simulink model "microarchi_router"  (R2015a)
settings: Solver=ode45  StartTime=0.0  StopTime=10.0  RelTol=1e-3
undefined symbols (not defined in the file or in its folder): des
(part 1 of 2)
settings Model: Creator=Nejib  LastModifiedBy=Nejib

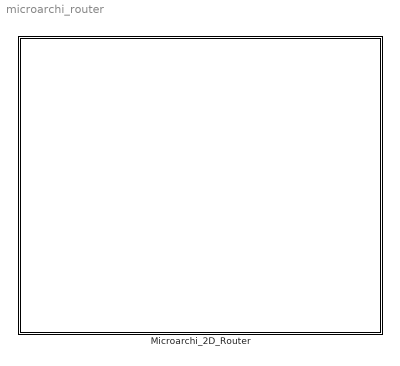
== system microarchi_router ==
  Microarchi_2D_Router : Subsystem  mask{C=16, P=1, ME_X=1, ME_Y=1, N_X=4, N_Y=4}
      mask prompts: C "FIFO size"; P "Clock period"; ME_X "X"; ME_Y "Y"; N_X "X"; N_Y "Y"

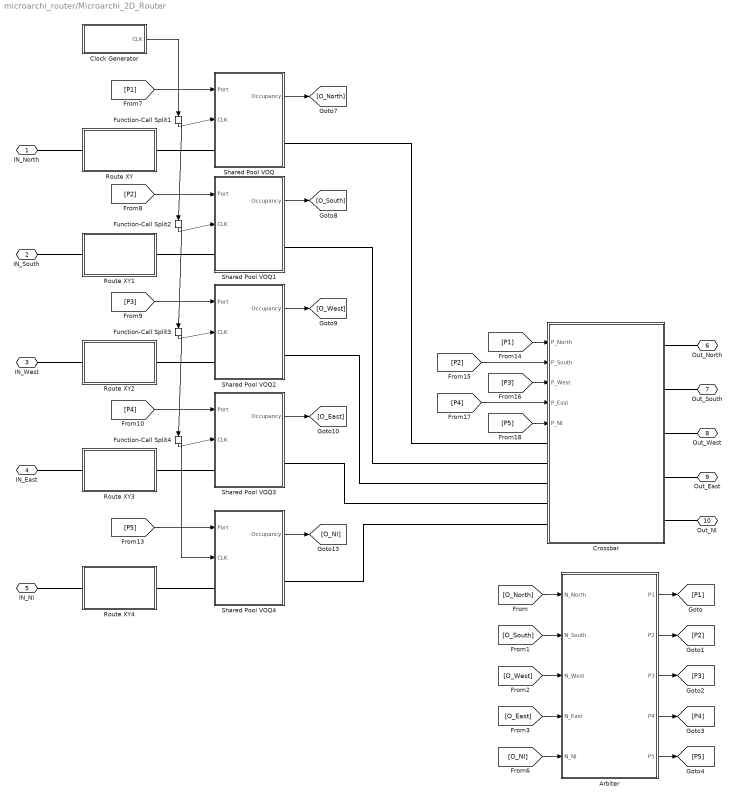
== system microarchi_router/Microarchi_2D_Router ==
  Arbiter : Subsystem  TreatAsAtomicUnit=on
  Clock Generator : Subsystem  mask{P=P}
      mask prompts: P "Period"
      mask DialogControl DescTextVar Prompt: Generates a perfectly periodic clock signal.
  Crossbar : Subsystem
  Function-Call Split{1..4} (4 alike) : FunctionCallSplit
  Route XY : Subsystem  mask{ME_X=ME_X, ME_Y=ME_Y, N_X=4, N_Y=4}
      mask prompts: ME_X "X"; ME_Y "Y"; N_X "X"; N_Y "Y"
  Route XY1 : Subsystem  mask{ME_X=ME_X, ME_Y=ME_Y, N_X=4, N_Y=4}
      mask prompts: ME_X "X"; ME_Y "Y"; N_X "X"; N_Y "Y"
  Route XY2 : Subsystem  mask{ME_X=ME_X, ME_Y=ME_Y, N_X=4, N_Y=4}
      mask prompts: ME_X "X"; ME_Y "Y"; N_X "X"; N_Y "Y"
  Route XY3 : Subsystem  mask{ME_X=ME_X, ME_Y=ME_Y, N_X=0, N_Y=0}
      mask prompts: ME_X "X"; ME_Y "Y"; N_X "X"; N_Y "Y"
  Route XY4 : Subsystem  mask{ME_X=ME_X, ME_Y=ME_Y, N_X=4, N_Y=4}
      mask prompts: ME_X "X"; ME_Y "Y"; N_X "X"; N_Y "Y"
  Shared Pool VOQ : Subsystem  mask{C=C}
      mask prompts: C "FIFO Size"
  Shared Pool VOQ1 : Subsystem  mask{C=C}
      mask prompts: C "FIFO Size"
  Shared Pool VOQ2 : Subsystem  mask{C=C}
      mask prompts: C "FIFO Size"
  Shared Pool VOQ3 : Subsystem  mask{C=C}
      mask prompts: C "FIFO Size"
  Shared Pool VOQ4 : Subsystem  mask{C=C}
      mask prompts: C "FIFO Size"
  IN_North : PMIOPort  Port=1  Side=Left
  IN_South : PMIOPort  Port=2  Side=Left
  IN_West : PMIOPort  Port=3  Side=Left
  IN_East : PMIOPort  Port=4  Side=Left
  IN_NI : PMIOPort  Port=5  Side=Left
  Out_North : PMIOPort  Port=6  Side=Right
  Out_South : PMIOPort  Port=7  Side=Right
  Out_West : PMIOPort  Port=8  Side=Right
  Out_East : PMIOPort  Port=9  Side=Right
  Out_NI : PMIOPort  Port=10  Side=Right
  wires:
  [O_NI] -> Arbiter/5(N_NI)
  [P5] -> Shared Pool VOQ4/1(Port)
  Arbiter/5(P5) -> [P5]
  [O_North] -> Arbiter/1(N_North)
  Shared Pool VOQ3/1(Occupancy) -> [O_East]
  Arbiter/3(P3) -> [P3]
  Arbiter/1(P1) -> [P1]
  [O_West] -> Arbiter/3(N_West)
  Shared Pool VOQ4/1(Occupancy) -> [O_NI]
  Arbiter/4(P4) -> [P4]
  Shared Pool VOQ2/1(Occupancy) -> [O_West]
  Shared Pool VOQ1/1(Occupancy) -> [O_South]
  [O_South] -> Arbiter/2(N_South)
  [P1] -> Shared Pool VOQ/1(Port)
  [O_East] -> Arbiter/4(N_East)
  Arbiter/2(P2) -> [P2]
  [P3] -> Shared Pool VOQ2/1(Port)
  [P4] -> Shared Pool VOQ3/1(Port)
  [P2] -> Shared Pool VOQ1/1(Port)
  Function-Call Split4/1 -> Shared Pool VOQ3/2(CLK)
  Function-Call Split3/2 -> Function-Call Split4/1
  Function-Call Split3/1 -> Shared Pool VOQ2/2(CLK)
  Function-Call Split2/2 -> Function-Call Split3/1
  Function-Call Split2/1 -> Shared Pool VOQ1/2(CLK)
  Function-Call Split1/2 -> Function-Call Split2/1
  Function-Call Split1/1 -> Shared Pool VOQ/2(CLK)
  Clock Generator/1(CLK) -> Function-Call Split1/1
  Shared Pool VOQ/1(Occupancy) -> [O_North]
  Function-Call Split4/2 -> Shared Pool VOQ4/2(CLK)
  [P1] -> Crossbar/1(P_North)
  [P2] -> Crossbar/2(P_South)
  [P3] -> Crossbar/3(P_West)
  [P4] -> Crossbar/4(P_East)
  [P5] -> Crossbar/5(P_NI)
  connections:
  Shared Pool VOQ/LConn1 -- Route XY/RConn1
  Shared Pool VOQ3/LConn1 -- Route XY3/RConn1
  Route XY1/LConn1 -- IN_South/RConn1
  IN_North/RConn1 -- Route XY/LConn1
  Route XY3/LConn1 -- IN_East/RConn1
  Route XY2/LConn1 -- IN_West/RConn1
  Route XY4/LConn1 -- IN_NI/RConn1
  Shared Pool VOQ1/LConn1 -- Route XY1/RConn1
  Shared Pool VOQ2/LConn1 -- Route XY2/RConn1
  Shared Pool VOQ4/LConn1 -- Route XY4/RConn1
  Out_North/RConn1 -- Crossbar/RConn1
  Out_South/RConn1 -- Crossbar/RConn2
  Out_West/RConn1 -- Crossbar/RConn3
  Out_East/RConn1 -- Crossbar/RConn4
  Out_NI/RConn1 -- Crossbar/RConn5
  Shared Pool VOQ4/RConn1 -- Crossbar/LConn5
  Shared Pool VOQ3/RConn1 -- Crossbar/LConn4
  Shared Pool VOQ2/RConn1 -- Crossbar/LConn3
  Shared Pool VOQ1/RConn1 -- Crossbar/LConn2
  Shared Pool VOQ/RConn1 -- Crossbar/LConn1

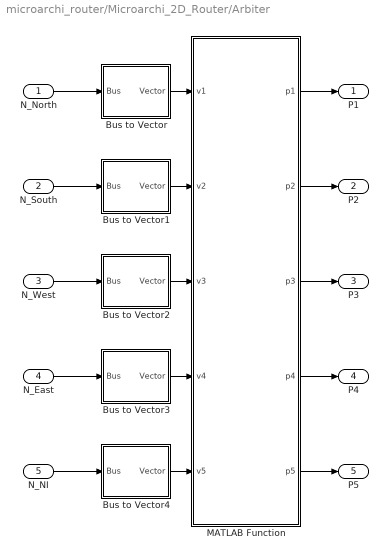
== system microarchi_router/Microarchi_2D_Router/Arbiter ==
  N_North : Inport
  N_South : Inport  Port=2
  N_West : Inport  Port=3
  N_East : Inport  Port=4
  N_NI : Inport  Port=5
  Bus to Vector : Subsystem
  Bus to Vector1 : Subsystem
  Bus to Vector2 : Subsystem
  Bus to Vector3 : Subsystem
  Bus to Vector4 : Subsystem
  MATLAB Function : MATLAB Function  TreatAsAtomicUnit=on
  P1 : Outport
  P2 : Outport  Port=2
  P3 : Outport  Port=3
  P4 : Outport  Port=4
  P5 : Outport  Port=5
  wires:
  N_North/1 -> Bus to Vector/1(Bus)
  N_South/1 -> Bus to Vector1/1(Bus)
  N_West/1 -> Bus to Vector2/1(Bus)
  N_East/1 -> Bus to Vector3/1(Bus)
  Bus to Vector2/1(Vector) -> MATLAB Function/3(v3)
  Bus to Vector1/1(Vector) -> MATLAB Function/2(v2)
  Bus to Vector3/1(Vector) -> MATLAB Function/4(v4)
  Bus to Vector/1(Vector) -> MATLAB Function/1(v1)
  MATLAB Function/2(p2) -> P2/1
  MATLAB Function/1(p1) -> P1/1
  MATLAB Function/3(p3) -> P3/1
  MATLAB Function/4(p4) -> P4/1
  MATLAB Function/5(p5) -> P5/1
  Bus to Vector4/1(Vector) -> MATLAB Function/5(v5)
  N_NI/1 -> Bus to Vector4/1(Bus)

== system microarchi_router/Microarchi_2D_Router/Clock Generator ==
  Time-Based Function-Call Generator : TimeBasedFunctionCallGenerator  Period=P  StatNumberOfEvents=on
      settings: OutputPortMap=o0,o1
  CLK : Outport
  wires:
  Time-Based Function-Call Generator/1 -> CLK/1

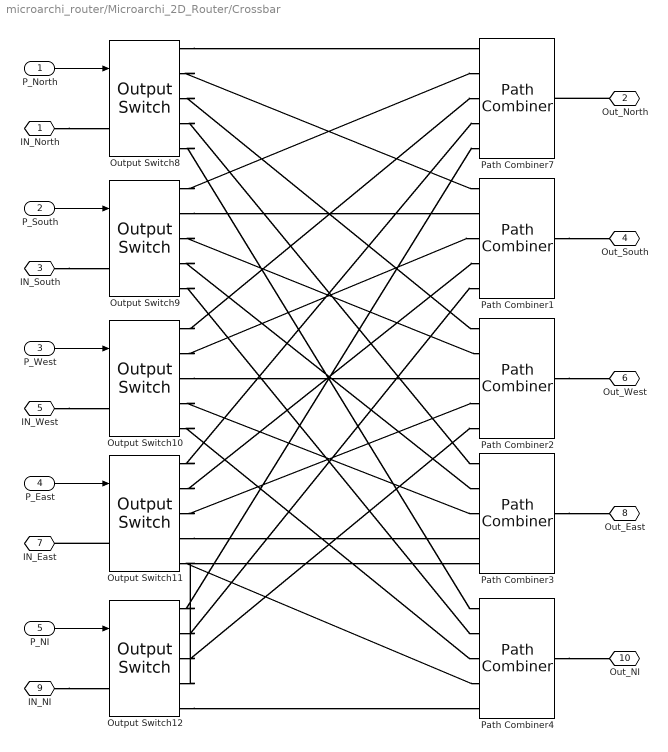
== system microarchi_router/Microarchi_2D_Router/Crossbar ==
  P_North : Inport
  P_South : Inport  Port=2
  P_West : Inport  Port=3
  P_East : Inport  Port=4
  P_NI : Inport  Port=5
  Output Switch{8..12} (5 alike) : OutputSwitch  NumberOutputPorts=5  SwitchingCriterion=From signal port p  AttributeName=RT
  Path Combiner{1..4,7} (5 alike) : PathCombiner  NumberInputPorts=5
  IN_North : PMIOPort  Port=1  Side=Left
  Out_North : PMIOPort  Port=2  Side=Right
  IN_South : PMIOPort  Port=3  Side=Left
  Out_South : PMIOPort  Port=4  Side=Right
  IN_West : PMIOPort  Port=5  Side=Left
  Out_West : PMIOPort  Port=6  Side=Right
  IN_East : PMIOPort  Port=7  Side=Left
  Out_East : PMIOPort  Port=8  Side=Right
  IN_NI : PMIOPort  Port=9  Side=Left
  Out_NI : PMIOPort  Port=10  Side=Right
  wires:
  P_North/1 -> Output Switch8/1
  P_South/1 -> Output Switch9/1
  P_West/1 -> Output Switch10/1
  P_East/1 -> Output Switch11/1
  P_NI/1 -> Output Switch12/1
  connections:
  IN_North/RConn1 -- Output Switch8/LConn1
  Path Combiner1/RConn1 -- Out_South/RConn1
  IN_South/RConn1 -- Output Switch9/LConn1
  Path Combiner2/RConn1 -- Out_West/RConn1
  IN_West/RConn1 -- Output Switch10/LConn1
  Path Combiner3/RConn1 -- Out_East/RConn1
  Output Switch11/LConn1 -- IN_East/RConn1
  IN_NI/RConn1 -- Output Switch12/LConn1
  Path Combiner4/RConn1 -- Out_NI/RConn1
  Output Switch8/RConn1 -- Path Combiner7/LConn1
  Out_North/RConn1 -- Path Combiner7/RConn1
  Output Switch9/RConn2 -- Path Combiner1/LConn2
  Output Switch10/RConn3 -- Path Combiner2/LConn3
  Output Switch11/RConn4 -- Path Combiner3/LConn4
  Output Switch12/RConn5 -- Path Combiner4/LConn5
  Output Switch8/RConn2 -- Path Combiner1/LConn1
  Output Switch8/RConn3 -- Path Combiner2/LConn1
  Output Switch8/RConn4 -- Path Combiner3/LConn1
  Output Switch8/RConn5 -- Path Combiner4/LConn1
  Output Switch9/RConn1 -- Path Combiner7/LConn2
  Output Switch9/RConn3 -- Path Combiner2/LConn2
  Output Switch9/RConn4 -- Path Combiner3/LConn2
  Output Switch9/RConn5 -- Path Combiner4/LConn2
  Output Switch10/RConn1 -- Path Combiner7/LConn3
  Output Switch10/RConn2 -- Path Combiner1/LConn3
  Output Switch10/RConn4 -- Path Combiner3/LConn3
  Output Switch10/RConn5 -- Path Combiner4/LConn3
  Output Switch11/RConn1 -- Path Combiner7/LConn4
  Output Switch11/RConn2 -- Path Combiner1/LConn4
  Output Switch11/RConn3 -- Path Combiner2/LConn4
  Output Switch11/RConn5 -- Path Combiner4/LConn4
  Output Switch12/RConn1 -- Path Combiner7/LConn5
  Output Switch12/RConn2 -- Path Combiner1/LConn5
  Output Switch12/RConn3 -- Path Combiner2/LConn5
  Output Switch12/RConn4 -- Path Combiner3/LConn5

== system microarchi_router/Microarchi_2D_Router/Route XY ==
  Attribute Function : Subsystem  LoadFcn=des.afb.attributefunction_support(gcb,'LoadFcn');  StartFcn=des.afb.attributefunction_support(gcb,'StartFcn');  mask(Attribute Function){OutputNamePrefix=out_}
      mask prompts: OutputNamePrefix "Prefix name"
      settings: CopyFcn=des.afb.attributefunction_support(gcb,'CopyFcn');  OpenFcn=des.afb.attributefunction_support(gcb,'OpenFcn');  ErrorFcn=des.afb.error_redirect
      mask Help: slhelp(gcbh)
      mask Display: image(des_iconLoad('attribFunction.jpg'),'center');
  Set Attribute : SetAttribute  AttributeName=IME_X|IME_Y  AttributeFrom=Dialog|Dialog  AttributeValue=ME_X|ME_Y  AttributeTreatAsVector=1|1  EvaluatedAttributeValue={ ME_X;ME_Y}
  Output : PMIOPort  Port=1  Side=Right
  Input : PMIOPort  Port=2  Side=Left
  connections:
  Attribute Function/RConn1 -- Output/RConn1
  Set Attribute/LConn1 -- Input/RConn1
  Set Attribute/RConn1 -- Attribute Function/LConn1

== system microarchi_router/Microarchi_2D_Router/Route XY1 ==
  Attribute Function : Subsystem  LoadFcn=des.afb.attributefunction_support(gcb,'LoadFcn');  StartFcn=des.afb.attributefunction_support(gcb,'StartFcn');  mask(Attribute Function){OutputNamePrefix=out_}
      mask prompts: OutputNamePrefix "Prefix name"
      settings: CopyFcn=des.afb.attributefunction_support(gcb,'CopyFcn');  OpenFcn=des.afb.attributefunction_support(gcb,'OpenFcn');  ErrorFcn=des.afb.error_redirect
      mask Help: slhelp(gcbh)
      mask Display: image(des_iconLoad('attribFunction.jpg'),'center');
  Set Attribute : SetAttribute  AttributeName=IME_X|IME_Y  AttributeFrom=Dialog|Dialog  AttributeValue=ME_X|ME_Y  AttributeTreatAsVector=1|1  EvaluatedAttributeValue={ ME_X;ME_Y}
  Output : PMIOPort  Port=1  Side=Right
  Input : PMIOPort  Port=2  Side=Left
  connections:
  Set Attribute/RConn1 -- Attribute Function/LConn1
  Set Attribute/LConn1 -- Input/RConn1
  Attribute Function/RConn1 -- Output/RConn1

== system microarchi_router/Microarchi_2D_Router/Route XY2 ==
  Attribute Function : Subsystem  LoadFcn=des.afb.attributefunction_support(gcb,'LoadFcn');  StartFcn=des.afb.attributefunction_support(gcb,'StartFcn');  mask(Attribute Function){OutputNamePrefix=out_}
      mask prompts: OutputNamePrefix "Prefix name"
      settings: CopyFcn=des.afb.attributefunction_support(gcb,'CopyFcn');  OpenFcn=des.afb.attributefunction_support(gcb,'OpenFcn');  ErrorFcn=des.afb.error_redirect
      mask Help: slhelp(gcbh)
      mask Display: image(des_iconLoad('attribFunction.jpg'),'center');
  Set Attribute : SetAttribute  AttributeName=IME_X|IME_Y  AttributeFrom=Dialog|Dialog  AttributeValue=ME_X|ME_Y  AttributeTreatAsVector=1|1  EvaluatedAttributeValue={ ME_X;ME_Y}
  Output : PMIOPort  Port=1  Side=Right
  Input : PMIOPort  Port=2  Side=Left
  connections:
  Attribute Function/RConn1 -- Output/RConn1
  Set Attribute/LConn1 -- Input/RConn1
  Set Attribute/RConn1 -- Attribute Function/LConn1

== system microarchi_router/Microarchi_2D_Router/Route XY3 ==
  Attribute Function : Subsystem  LoadFcn=des.afb.attributefunction_support(gcb,'LoadFcn');  StartFcn=des.afb.attributefunction_support(gcb,'StartFcn');  mask(Attribute Function){OutputNamePrefix=out_}
      mask prompts: OutputNamePrefix "Prefix name"
      settings: CopyFcn=des.afb.attributefunction_support(gcb,'CopyFcn');  OpenFcn=des.afb.attributefunction_support(gcb,'OpenFcn');  ErrorFcn=des.afb.error_redirect
      mask Help: slhelp(gcbh)
      mask Display: image(des_iconLoad('attribFunction.jpg'),'center');
  Set Attribute : SetAttribute  AttributeName=IME_X|IME_Y  AttributeFrom=Dialog|Dialog  AttributeValue=ME_X|ME_Y  AttributeTreatAsVector=1|1  EvaluatedAttributeValue={ ME_X;ME_Y}
  Output : PMIOPort  Port=1  Side=Right
  Input : PMIOPort  Port=2  Side=Left
  connections:
  Set Attribute/RConn1 -- Attribute Function/LConn1
  Set Attribute/LConn1 -- Input/RConn1
  Attribute Function/RConn1 -- Output/RConn1

== system microarchi_router/Microarchi_2D_Router/Route XY4 ==
  Attribute Function : Subsystem  LoadFcn=des.afb.attributefunction_support(gcb,'LoadFcn');  StartFcn=des.afb.attributefunction_support(gcb,'StartFcn');  mask(Attribute Function){OutputNamePrefix=out_}
      mask prompts: OutputNamePrefix "Prefix name"
      settings: CopyFcn=des.afb.attributefunction_support(gcb,'CopyFcn');  OpenFcn=des.afb.attributefunction_support(gcb,'OpenFcn');  ErrorFcn=des.afb.error_redirect
      mask Help: slhelp(gcbh)
      mask Display: image(des_iconLoad('attribFunction.jpg'),'center');
  Set Attribute : SetAttribute  AttributeName=IME_X|IME_Y  AttributeFrom=Dialog|Dialog  AttributeValue=ME_X|ME_Y  AttributeTreatAsVector=1|1  EvaluatedAttributeValue={ ME_X;ME_Y}
  Output : PMIOPort  Port=1  Side=Right
  Input : PMIOPort  Port=2  Side=Left
  connections:
  Attribute Function/RConn1 -- Output/RConn1
  Set Attribute/LConn1 -- Input/RConn1
  Set Attribute/RConn1 -- Attribute Function/LConn1

== system microarchi_router/Microarchi_2D_Router/Shared Pool VOQ ==
  Port : Inport
  CLK : Inport  Port=2
  Get Attribute : GetAttribute  AttributeName=RT|DST_X|DST_Y  AttributeMissing=Error|Error|Error  AttributeDefaultValue=1|1|1  AttributeTreatAsVector=1|1|1  AttributeSendTiming=After entity departure|After entity departure|After entity departure  EvaluatedDefaultAttributeValue={ [];[];[]}
      settings: OutputPortMap=o1,o2,o3
  Mux : Mux  Inputs=6
      settings: DisplayOption=signals
  voq : Subsystem
  Input : PMIOPort  Port=1  Side=Left
  Output : PMIOPort  Port=2  Side=Right
  Occupancy : Outport
  wires:
  Port/1 -> voq/1(Port)
  Mux/1 -> Occupancy/1
  voq/6(n5) -> Mux/6
  voq/1(n) -> Mux/1
  voq/5(n4) -> Mux/5
  voq/4(n3) -> Mux/4
  voq/2(n1) -> Mux/2
  voq/3(n2) -> Mux/3
  CLK/1 -> voq/2(CLK)
  connections:
  voq/RConn1 -- Output/RConn1
  Input/RConn1 -- Get Attribute/LConn1
  Get Attribute/RConn1 -- voq/LConn1

== system microarchi_router/Microarchi_2D_Router/Shared Pool VOQ1 ==
  Port : Inport
  CLK : Inport  Port=2
  Get Attribute : GetAttribute  AttributeName=RT|DST_X|DST_Y  AttributeMissing=Error|Error|Error  AttributeDefaultValue=1|1|1  AttributeTreatAsVector=1|1|1  AttributeSendTiming=After entity departure|After entity departure|After entity departure  EvaluatedDefaultAttributeValue={ [];[];[]}
      settings: OutputPortMap=o1,o2,o3
  Mux : Mux  Inputs=6
      settings: DisplayOption=signals
  voq : Subsystem
  Input : PMIOPort  Port=1  Side=Left
  Output : PMIOPort  Port=2  Side=Right
  Occupancy : Outport
  wires:
  CLK/1 -> voq/2(CLK)
  voq/3(n2) -> Mux/3
  voq/2(n1) -> Mux/2
  voq/4(n3) -> Mux/4
  voq/5(n4) -> Mux/5
  voq/1(n) -> Mux/1
  voq/6(n5) -> Mux/6
  Mux/1 -> Occupancy/1
  Port/1 -> voq/1(Port)
  connections:
  Get Attribute/RConn1 -- voq/LConn1
  Input/RConn1 -- Get Attribute/LConn1
  voq/RConn1 -- Output/RConn1

== system microarchi_router/Microarchi_2D_Router/Shared Pool VOQ2 ==
  Port : Inport
  CLK : Inport  Port=2
  Get Attribute : GetAttribute  AttributeName=RT|DST_X|DST_Y  AttributeMissing=Error|Error|Error  AttributeDefaultValue=1|1|1  AttributeTreatAsVector=1|1|1  AttributeSendTiming=After entity departure|After entity departure|After entity departure  EvaluatedDefaultAttributeValue={ [];[];[]}
      settings: OutputPortMap=o1,o2,o3
  Mux : Mux  Inputs=6
      settings: DisplayOption=signals
  voq : Subsystem
  Input : PMIOPort  Port=1  Side=Left
  Output : PMIOPort  Port=2  Side=Right
  Occupancy : Outport
  wires:
  Port/1 -> voq/1(Port)
  Mux/1 -> Occupancy/1
  voq/6(n5) -> Mux/6
  voq/1(n) -> Mux/1
  voq/5(n4) -> Mux/5
  voq/4(n3) -> Mux/4
  voq/2(n1) -> Mux/2
  voq/3(n2) -> Mux/3
  CLK/1 -> voq/2(CLK)
  connections:
  voq/RConn1 -- Output/RConn1
  Input/RConn1 -- Get Attribute/LConn1
  Get Attribute/RConn1 -- voq/LConn1

== system microarchi_router/Microarchi_2D_Router/Shared Pool VOQ3 ==
  Port : Inport
  CLK : Inport  Port=2
  Get Attribute : GetAttribute  AttributeName=RT|DST_X|DST_Y  AttributeMissing=Error|Error|Error  AttributeDefaultValue=1|1|1  AttributeTreatAsVector=1|1|1  AttributeSendTiming=After entity departure|After entity departure|After entity departure  EvaluatedDefaultAttributeValue={ [];[];[]}
      settings: OutputPortMap=o1,o2,o3
  Mux : Mux  Inputs=6
      settings: DisplayOption=signals
  voq : Subsystem
  Input : PMIOPort  Port=1  Side=Left
  Output : PMIOPort  Port=2  Side=Right
  Occupancy : Outport
  wires:
  CLK/1 -> voq/2(CLK)
  voq/3(n2) -> Mux/3
  voq/2(n1) -> Mux/2
  voq/4(n3) -> Mux/4
  voq/5(n4) -> Mux/5
  voq/1(n) -> Mux/1
  voq/6(n5) -> Mux/6
  Mux/1 -> Occupancy/1
  Port/1 -> voq/1(Port)
  connections:
  Get Attribute/RConn1 -- voq/LConn1
  Input/RConn1 -- Get Attribute/LConn1
  voq/RConn1 -- Output/RConn1

== system microarchi_router/Microarchi_2D_Router/Shared Pool VOQ4 ==
  Port : Inport
  CLK : Inport  Port=2
  Get Attribute : GetAttribute  AttributeName=RT|DST_X|DST_Y  AttributeMissing=Error|Error|Error  AttributeDefaultValue=1|1|1  AttributeTreatAsVector=1|1|1  AttributeSendTiming=After entity departure|After entity departure|After entity departure  EvaluatedDefaultAttributeValue={ [];[];[]}
      settings: OutputPortMap=o1,o2,o3
  Mux : Mux  Inputs=6
      settings: DisplayOption=signals
  voq : Subsystem
  Input : PMIOPort  Port=1  Side=Left
  Output : PMIOPort  Port=2  Side=Right
  Occupancy : Outport
  wires:
  Port/1 -> voq/1(Port)
  Mux/1 -> Occupancy/1
  voq/6(n5) -> Mux/6
  voq/1(n) -> Mux/1
  voq/5(n4) -> Mux/5
  voq/4(n3) -> Mux/4
  voq/2(n1) -> Mux/2
  voq/3(n2) -> Mux/3
  CLK/1 -> voq/2(CLK)
  connections:
  voq/RConn1 -- Output/RConn1
  Input/RConn1 -- Get Attribute/LConn1
  Get Attribute/RConn1 -- voq/LConn1

== system microarchi_router/Microarchi_2D_Router/Arbiter/Bus to Vector ==
  Bus : Inport
  Demux : Demux  Outputs=6
  Vector Concatenate : Concatenate  NumInputs=6
  Vector : Outport
  wires:
  Demux/1 -> Vector Concatenate/1
  Bus/1 -> Demux/1
  Vector Concatenate/1 -> Vector/1
  Demux/2 -> Vector Concatenate/2
  Demux/3 -> Vector Concatenate/3
  Demux/4 -> Vector Concatenate/4
  Demux/5 -> Vector Concatenate/5
  Demux/6 -> Vector Concatenate/6

== system microarchi_router/Microarchi_2D_Router/Arbiter/Bus to Vector1 ==
  Bus : Inport
  Demux : Demux  Outputs=6
  Vector Concatenate : Concatenate  NumInputs=6
  Vector : Outport
  wires:
  Demux/6 -> Vector Concatenate/6
  Demux/5 -> Vector Concatenate/5
  Demux/4 -> Vector Concatenate/4
  Demux/3 -> Vector Concatenate/3
  Demux/2 -> Vector Concatenate/2
  Vector Concatenate/1 -> Vector/1
  Bus/1 -> Demux/1
  Demux/1 -> Vector Concatenate/1

== system microarchi_router/Microarchi_2D_Router/Arbiter/Bus to Vector2 ==
  Bus : Inport
  Demux : Demux  Outputs=6
  Vector Concatenate : Concatenate  NumInputs=6
  Vector : Outport
  wires:
  Demux/1 -> Vector Concatenate/1
  Bus/1 -> Demux/1
  Vector Concatenate/1 -> Vector/1
  Demux/2 -> Vector Concatenate/2
  Demux/3 -> Vector Concatenate/3
  Demux/4 -> Vector Concatenate/4
  Demux/5 -> Vector Concatenate/5
  Demux/6 -> Vector Concatenate/6

== system microarchi_router/Microarchi_2D_Router/Arbiter/Bus to Vector3 ==
  Bus : Inport
  Demux : Demux  Outputs=6
  Vector Concatenate : Concatenate  NumInputs=6
  Vector : Outport
  wires:
  Demux/6 -> Vector Concatenate/6
  Demux/5 -> Vector Concatenate/5
  Demux/4 -> Vector Concatenate/4
  Demux/3 -> Vector Concatenate/3
  Demux/2 -> Vector Concatenate/2
  Vector Concatenate/1 -> Vector/1
  Bus/1 -> Demux/1
  Demux/1 -> Vector Concatenate/1

== system microarchi_router/Microarchi_2D_Router/Arbiter/Bus to Vector4 ==
  Bus : Inport
  Demux : Demux  Outputs=6
  Vector Concatenate : Concatenate  NumInputs=6
  Vector : Outport
  wires:
  Demux/1 -> Vector Concatenate/1
  Bus/1 -> Demux/1
  Vector Concatenate/1 -> Vector/1
  Demux/2 -> Vector Concatenate/2
  Demux/3 -> Vector Concatenate/3
  Demux/4 -> Vector Concatenate/4
  Demux/5 -> Vector Concatenate/5
  Demux/6 -> Vector Concatenate/6

== system microarchi_router/Microarchi_2D_Router/Route XY/Attribute Function ==
  MATLAB Function : MATLAB Function  TreatAsAtomicUnit=on
  __DMLF__EDE2FCE__ : EntityDepartureFunctionCallGenerator  TimingFunctionCallF1=Before entity departure  IsInsideAFB=on
  __DMLF__GA__ : GetAttribute  AttributeName=DST_X|DST_Y|IME_X|IME_Y  AttributeMissing=Error|Error|Error|Error  AttributeDefaultValue=1|1|1|1  AttributeTreatAsVector=1|1|1|1  AttributeSendTiming=Before entity departure|Before entity departure|Before entity departure|Before entity departure  EvaluatedDefaultAttributeValue={ [];[];[];[]}  IsInsideAFB=on
      settings: OutputPortMap=o1,o2,o3,o4
  __DMLF__SA__ : SetAttribute  AttributeName=RT  AttributeFrom=Signal port  EvaluatedAttributeValue={ []}  IsInsideAFB=on
  IN : PMIOPort  Port=1  Side=Left
  OUT : PMIOPort  Port=2  Side=Right
  wires:
  __DMLF__EDE2FCE__/1 -> MATLAB Function/Trigger
  __DMLF__GA__/1 -> MATLAB Function/1(DST_X)
  __DMLF__GA__/2 -> MATLAB Function/2(DST_Y)
  __DMLF__GA__/3 -> MATLAB Function/3(IME_X)
  __DMLF__GA__/4 -> MATLAB Function/4(IME_Y)
  MATLAB Function/1(out_RT) -> __DMLF__SA__/1
  connections:
  __DMLF__SA__/LConn1 -- __DMLF__EDE2FCE__/RConn1
  __DMLF__GA__/RConn1 -- __DMLF__EDE2FCE__/LConn1
  IN/RConn1 -- __DMLF__GA__/LConn1
  __DMLF__SA__/RConn1 -- OUT/RConn1

== system microarchi_router/Microarchi_2D_Router/Route XY1/Attribute Function ==
  MATLAB Function : MATLAB Function  TreatAsAtomicUnit=on
  __DMLF__EDE2FCE__ : EntityDepartureFunctionCallGenerator  TimingFunctionCallF1=Before entity departure  IsInsideAFB=on
  __DMLF__GA__ : GetAttribute  AttributeName=DST_X|DST_Y|IME_X|IME_Y  AttributeMissing=Error|Error|Error|Error  AttributeDefaultValue=1|1|1|1  AttributeTreatAsVector=1|1|1|1  AttributeSendTiming=Before entity departure|Before entity departure|Before entity departure|Before entity departure  EvaluatedDefaultAttributeValue={ [];[];[];[]}  IsInsideAFB=on
      settings: OutputPortMap=o1,o2,o3,o4
  __DMLF__SA__ : SetAttribute  AttributeName=RT  AttributeFrom=Signal port  EvaluatedAttributeValue={ []}  IsInsideAFB=on
  IN : PMIOPort  Port=1  Side=Left
  OUT : PMIOPort  Port=2  Side=Right
  wires:
  __DMLF__EDE2FCE__/1 -> MATLAB Function/Trigger
  __DMLF__GA__/1 -> MATLAB Function/1(DST_X)
  __DMLF__GA__/2 -> MATLAB Function/2(DST_Y)
  __DMLF__GA__/3 -> MATLAB Function/3(IME_X)
  __DMLF__GA__/4 -> MATLAB Function/4(IME_Y)
  MATLAB Function/1(out_RT) -> __DMLF__SA__/1
  connections:
  __DMLF__SA__/RConn1 -- OUT/RConn1
  IN/RConn1 -- __DMLF__GA__/LConn1
  __DMLF__GA__/RConn1 -- __DMLF__EDE2FCE__/LConn1
  __DMLF__SA__/LConn1 -- __DMLF__EDE2FCE__/RConn1

== system microarchi_router/Microarchi_2D_Router/Route XY2/Attribute Function ==
  MATLAB Function : MATLAB Function  TreatAsAtomicUnit=on
  __DMLF__EDE2FCE__ : EntityDepartureFunctionCallGenerator  TimingFunctionCallF1=Before entity departure  IsInsideAFB=on
  __DMLF__GA__ : GetAttribute  AttributeName=DST_X|DST_Y|IME_X|IME_Y  AttributeMissing=Error|Error|Error|Error  AttributeDefaultValue=1|1|1|1  AttributeTreatAsVector=1|1|1|1  AttributeSendTiming=Before entity departure|Before entity departure|Before entity departure|Before entity departure  EvaluatedDefaultAttributeValue={ [];[];[];[]}  IsInsideAFB=on
      settings: OutputPortMap=o1,o2,o3,o4
  __DMLF__SA__ : SetAttribute  AttributeName=RT  AttributeFrom=Signal port  EvaluatedAttributeValue={ []}  IsInsideAFB=on
  IN : PMIOPort  Port=1  Side=Left
  OUT : PMIOPort  Port=2  Side=Right
  wires:
  __DMLF__EDE2FCE__/1 -> MATLAB Function/Trigger
  __DMLF__GA__/1 -> MATLAB Function/1(DST_X)
  __DMLF__GA__/2 -> MATLAB Function/2(DST_Y)
  __DMLF__GA__/3 -> MATLAB Function/3(IME_X)
  __DMLF__GA__/4 -> MATLAB Function/4(IME_Y)
  MATLAB Function/1(out_RT) -> __DMLF__SA__/1
  connections:
  __DMLF__SA__/LConn1 -- __DMLF__EDE2FCE__/RConn1
  __DMLF__GA__/RConn1 -- __DMLF__EDE2FCE__/LConn1
  IN/RConn1 -- __DMLF__GA__/LConn1
  __DMLF__SA__/RConn1 -- OUT/RConn1

== system microarchi_router/Microarchi_2D_Router/Route XY3/Attribute Function ==
  MATLAB Function : MATLAB Function  TreatAsAtomicUnit=on
  __DMLF__EDE2FCE__ : EntityDepartureFunctionCallGenerator  TimingFunctionCallF1=Before entity departure  IsInsideAFB=on
  __DMLF__GA__ : GetAttribute  AttributeName=DST_X|DST_Y|IME_X|IME_Y  AttributeMissing=Error|Error|Error|Error  AttributeDefaultValue=1|1|1|1  AttributeTreatAsVector=1|1|1|1  AttributeSendTiming=Before entity departure|Before entity departure|Before entity departure|Before entity departure  EvaluatedDefaultAttributeValue={ [];[];[];[]}  IsInsideAFB=on
      settings: OutputPortMap=o1,o2,o3,o4
  __DMLF__SA__ : SetAttribute  AttributeName=RT  AttributeFrom=Signal port  EvaluatedAttributeValue={ []}  IsInsideAFB=on
  IN : PMIOPort  Port=1  Side=Left
  OUT : PMIOPort  Port=2  Side=Right
  wires:
  __DMLF__EDE2FCE__/1 -> MATLAB Function/Trigger
  __DMLF__GA__/1 -> MATLAB Function/1(DST_X)
  __DMLF__GA__/2 -> MATLAB Function/2(DST_Y)
  __DMLF__GA__/3 -> MATLAB Function/3(IME_X)
  __DMLF__GA__/4 -> MATLAB Function/4(IME_Y)
  MATLAB Function/1(out_RT) -> __DMLF__SA__/1
  connections:
  __DMLF__SA__/RConn1 -- OUT/RConn1
  IN/RConn1 -- __DMLF__GA__/LConn1
  __DMLF__GA__/RConn1 -- __DMLF__EDE2FCE__/LConn1
  __DMLF__SA__/LConn1 -- __DMLF__EDE2FCE__/RConn1

== system microarchi_router/Microarchi_2D_Router/Route XY4/Attribute Function ==
  MATLAB Function : MATLAB Function  TreatAsAtomicUnit=on
  __DMLF__EDE2FCE__ : EntityDepartureFunctionCallGenerator  TimingFunctionCallF1=Before entity departure  IsInsideAFB=on
  __DMLF__GA__ : GetAttribute  AttributeName=DST_X|DST_Y|IME_X|IME_Y  AttributeMissing=Error|Error|Error|Error  AttributeDefaultValue=1|1|1|1  AttributeTreatAsVector=1|1|1|1  AttributeSendTiming=Before entity departure|Before entity departure|Before entity departure|Before entity departure  EvaluatedDefaultAttributeValue={ [];[];[];[]}  IsInsideAFB=on
      settings: OutputPortMap=o1,o2,o3,o4
  __DMLF__SA__ : SetAttribute  AttributeName=RT  AttributeFrom=Signal port  EvaluatedAttributeValue={ []}  IsInsideAFB=on
  IN : PMIOPort  Port=1  Side=Left
  OUT : PMIOPort  Port=2  Side=Right
  wires:
  __DMLF__EDE2FCE__/1 -> MATLAB Function/Trigger
  __DMLF__GA__/1 -> MATLAB Function/1(DST_X)
  __DMLF__GA__/2 -> MATLAB Function/2(DST_Y)
  __DMLF__GA__/3 -> MATLAB Function/3(IME_X)
  __DMLF__GA__/4 -> MATLAB Function/4(IME_Y)
  MATLAB Function/1(out_RT) -> __DMLF__SA__/1
  connections:
  __DMLF__SA__/LConn1 -- __DMLF__EDE2FCE__/RConn1
  __DMLF__GA__/RConn1 -- __DMLF__EDE2FCE__/LConn1
  IN/RConn1 -- __DMLF__GA__/LConn1
  __DMLF__SA__/RConn1 -- OUT/RConn1

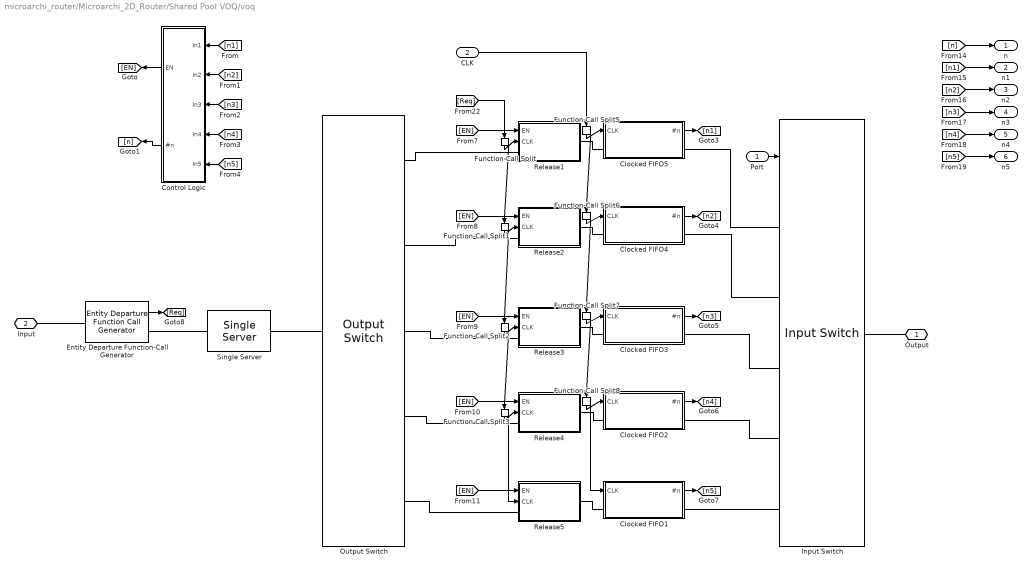
== system microarchi_router/Microarchi_2D_Router/Shared Pool VOQ/voq ==
  Port : Inport
  CLK : Inport  Port=2
  Clocked FIFO1 : Subsystem  mask{E=0, S=0, F=C}
      mask prompts: E "Clock Period (s)"; S "Standard Deviation"; F "FIFO capacity"
  Clocked FIFO2 : Subsystem  mask{E=0, S=0, F=C}
      mask prompts: E "Clock Period (s)"; S "Standard Deviation"; F "FIFO capacity"
  Clocked FIFO3 : Subsystem  mask{E=0, S=0, F=C}
      mask prompts: E "Clock Period (s)"; S "Standard Deviation"; F "FIFO capacity"
  Clocked FIFO4 : Subsystem  mask{E=0, S=0, F=C}
      mask prompts: E "Clock Period (s)"; S "Standard Deviation"; F "FIFO capacity"
  Clocked FIFO5 : Subsystem  mask{E=0, S=0, F=C}
      mask prompts: E "Clock Period (s)"; S "Standard Deviation"; F "FIFO capacity"
  Control Logic : Subsystem  TreatAsAtomicUnit=on
  Entity Departure Function-Call Generator : EntityDepartureFunctionCallGenerator
  Function-Call Split{,1..3,5..8} (8 alike) : FunctionCallSplit
  Input Switch : InputSwitch  NumberInputPorts=5  SwitchingCriterion=From signal port p
  Output Switch : OutputSwitch  NumberOutputPorts=5  SwitchingCriterion=From attribute  AttributeName=RT
  Release1 : Subsystem
  Release2 : Subsystem
  Release3 : Subsystem
  Release4 : Subsystem
  Release5 : Subsystem
  Single Server : SingleServer  ServiceTime=0
  Output : PMIOPort  Port=1  Side=Right
  Input : PMIOPort  Port=2  Side=Left
  n : Outport
  n1 : Outport  Port=2
  n2 : Outport  Port=3
  n3 : Outport  Port=4
  n4 : Outport  Port=5
  n5 : Outport  Port=6
  wires:
  Port/1 -> Input Switch/1
  [n1] -> Control Logic/1(In1)
  [n2] -> Control Logic/2(In2)
  [n3] -> Control Logic/3(In3)
  [n5] -> Control Logic/5(In5)
  [n4] -> Control Logic/4(In4)
  Control Logic/1(EN) -> [EN]
  Control Logic/2(#n) -> [n]
  Clocked FIFO5/1(#n) -> [n1]
  Clocked FIFO4/1(#n) -> [n2]
  Clocked FIFO3/1(#n) -> [n3]
  Clocked FIFO2/1(#n) -> [n4]
  Clocked FIFO1/1(#n) -> [n5]
  [EN] -> Release5/1(EN)
  [EN] -> Release4/1(EN)
  [EN] -> Release3/1(EN)
  [EN] -> Release2/1(EN)
  [EN] -> Release1/1(EN)
  [n] -> n/1
  [n1] -> n1/1
  [n2] -> n2/1
  [n3] -> n3/1
  [n4] -> n4/1
  [n5] -> n5/1
  Entity Departure Function-Call Generator/1 -> [Req]
  Function-Call Split8/1 -> Clocked FIFO2/1(CLK)
  Function-Call Split7/2 -> Function-Call Split8/1
  Function-Call Split7/1 -> Clocked FIFO3/1(CLK)
  Function-Call Split6/2 -> Function-Call Split7/1
  Function-Call Split6/1 -> Clocked FIFO4/1(CLK)
  Function-Call Split5/2 -> Function-Call Split6/1
  Function-Call Split5/1 -> Clocked FIFO5/1(CLK)
  CLK/1 -> Function-Call Split5/1
  Function-Call Split/1 -> Release1/2(CLK)
  Function-Call Split1/1 -> Release2/2(CLK)
  Function-Call Split2/1 -> Release3/2(CLK)
  Function-Call Split3/1 -> Release4/2(CLK)
  Function-Call Split2/2 -> Function-Call Split3/1
  Function-Call Split1/2 -> Function-Call Split2/1
  Function-Call Split/2 -> Function-Call Split1/1
  [Req] -> Function-Call Split/1
  Function-Call Split8/2 -> Clocked FIFO1/1(CLK)
  Function-Call Split3/2 -> Release5/2(CLK)
  connections:
  Clocked FIFO5/LConn1 -- Release1/RConn1
  Input/RConn1 -- Entity Departure Function-Call Generator/LConn1
  Release3/RConn1 -- Clocked FIFO3/LConn1
  Release4/RConn1 -- Clocked FIFO2/LConn1
  Release2/RConn1 -- Clocked FIFO4/LConn1
  Release3/LConn1 -- Output Switch/RConn3
  Release2/LConn1 -- Output Switch/RConn2
  Release4/LConn1 -- Output Switch/RConn4
  Output Switch/RConn1 -- Release1/LConn1
  Input Switch/RConn1 -- Output/RConn1
  Release5/RConn1 -- Clocked FIFO1/LConn1
  Release5/LConn1 -- Output Switch/RConn5
  Clocked FIFO5/RConn1 -- Input Switch/LConn1
  Clocked FIFO4/RConn1 -- Input Switch/LConn2
  Clocked FIFO3/RConn1 -- Input Switch/LConn3
  Clocked FIFO2/RConn1 -- Input Switch/LConn4
  Clocked FIFO1/RConn1 -- Input Switch/LConn5
  Entity Departure Function-Call Generator/RConn1 -- Single Server/LConn1
  Single Server/RConn1 -- Output Switch/LConn1

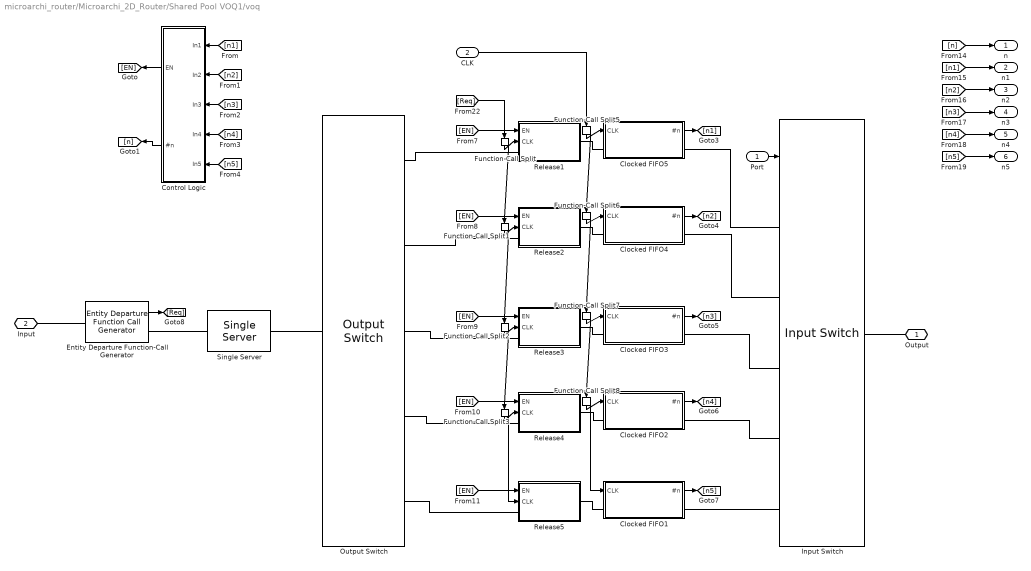
== system microarchi_router/Microarchi_2D_Router/Shared Pool VOQ1/voq ==
  Port : Inport
  CLK : Inport  Port=2
  Clocked FIFO1 : Subsystem  mask{E=0, S=0, F=C}
      mask prompts: E "Clock Period (s)"; S "Standard Deviation"; F "FIFO capacity"
  Clocked FIFO2 : Subsystem  mask{E=0, S=0, F=C}
      mask prompts: E "Clock Period (s)"; S "Standard Deviation"; F "FIFO capacity"
  Clocked FIFO3 : Subsystem  mask{E=0, S=0, F=C}
      mask prompts: E "Clock Period (s)"; S "Standard Deviation"; F "FIFO capacity"
  Clocked FIFO4 : Subsystem  mask{E=0, S=0, F=C}
      mask prompts: E "Clock Period (s)"; S "Standard Deviation"; F "FIFO capacity"
  Clocked FIFO5 : Subsystem  mask{E=0, S=0, F=C}
      mask prompts: E "Clock Period (s)"; S "Standard Deviation"; F "FIFO capacity"
  Control Logic : Subsystem  TreatAsAtomicUnit=on
  Entity Departure Function-Call Generator : EntityDepartureFunctionCallGenerator
  Function-Call Split{,1..3,5..8} (8 alike) : FunctionCallSplit
  Input Switch : InputSwitch  NumberInputPorts=5  SwitchingCriterion=From signal port p
  Output Switch : OutputSwitch  NumberOutputPorts=5  SwitchingCriterion=From attribute  AttributeName=RT
  Release1 : Subsystem
  Release2 : Subsystem
  Release3 : Subsystem
  Release4 : Subsystem
  Release5 : Subsystem
  Single Server : SingleServer  ServiceTime=0
  Output : PMIOPort  Port=1  Side=Right
  Input : PMIOPort  Port=2  Side=Left
  n : Outport
  n1 : Outport  Port=2
  n2 : Outport  Port=3
  n3 : Outport  Port=4
  n4 : Outport  Port=5
  n5 : Outport  Port=6
  wires:
  Function-Call Split3/2 -> Release5/2(CLK)
  Function-Call Split8/2 -> Clocked FIFO1/1(CLK)
  [Req] -> Function-Call Split/1
  Function-Call Split/2 -> Function-Call Split1/1
  Function-Call Split1/2 -> Function-Call Split2/1
  Function-Call Split2/2 -> Function-Call Split3/1
  Function-Call Split3/1 -> Release4/2(CLK)
  Function-Call Split2/1 -> Release3/2(CLK)
  Function-Call Split1/1 -> Release2/2(CLK)
  Function-Call Split/1 -> Release1/2(CLK)
  CLK/1 -> Function-Call Split5/1
  Function-Call Split5/1 -> Clocked FIFO5/1(CLK)
  Function-Call Split5/2 -> Function-Call Split6/1
  Function-Call Split6/1 -> Clocked FIFO4/1(CLK)
  Function-Call Split6/2 -> Function-Call Split7/1
  Function-Call Split7/1 -> Clocked FIFO3/1(CLK)
  Function-Call Split7/2 -> Function-Call Split8/1
  Function-Call Split8/1 -> Clocked FIFO2/1(CLK)
  Entity Departure Function-Call Generator/1 -> [Req]
  [n5] -> n5/1
  [n4] -> n4/1
  [n3] -> n3/1
  [n2] -> n2/1
  [n1] -> n1/1
  [n] -> n/1
  [EN] -> Release1/1(EN)
  [EN] -> Release2/1(EN)
  [EN] -> Release3/1(EN)
  [EN] -> Release4/1(EN)
  [EN] -> Release5/1(EN)
  Clocked FIFO1/1(#n) -> [n5]
  Clocked FIFO2/1(#n) -> [n4]
  Clocked FIFO3/1(#n) -> [n3]
  Clocked FIFO4/1(#n) -> [n2]
  Clocked FIFO5/1(#n) -> [n1]
  Control Logic/2(#n) -> [n]
  Control Logic/1(EN) -> [EN]
  [n4] -> Control Logic/4(In4)
  [n5] -> Control Logic/5(In5)
  [n3] -> Control Logic/3(In3)
  [n2] -> Control Logic/2(In2)
  [n1] -> Control Logic/1(In1)
  Port/1 -> Input Switch/1
  connections:
  Single Server/RConn1 -- Output Switch/LConn1
  Entity Departure Function-Call Generator/RConn1 -- Single Server/LConn1
  Clocked FIFO1/RConn1 -- Input Switch/LConn5
  Clocked FIFO2/RConn1 -- Input Switch/LConn4
  Clocked FIFO3/RConn1 -- Input Switch/LConn3
  Clocked FIFO4/RConn1 -- Input Switch/LConn2
  Clocked FIFO5/RConn1 -- Input Switch/LConn1
  Release5/LConn1 -- Output Switch/RConn5
  Release5/RConn1 -- Clocked FIFO1/LConn1
  Input Switch/RConn1 -- Output/RConn1
  Output Switch/RConn1 -- Release1/LConn1
  Release4/LConn1 -- Output Switch/RConn4
  Release2/LConn1 -- Output Switch/RConn2
  Release3/LConn1 -- Output Switch/RConn3
  Release2/RConn1 -- Clocked FIFO4/LConn1
  Release4/RConn1 -- Clocked FIFO2/LConn1
  Release3/RConn1 -- Clocked FIFO3/LConn1
  Input/RConn1 -- Entity Departure Function-Call Generator/LConn1
  Clocked FIFO5/LConn1 -- Release1/RConn1

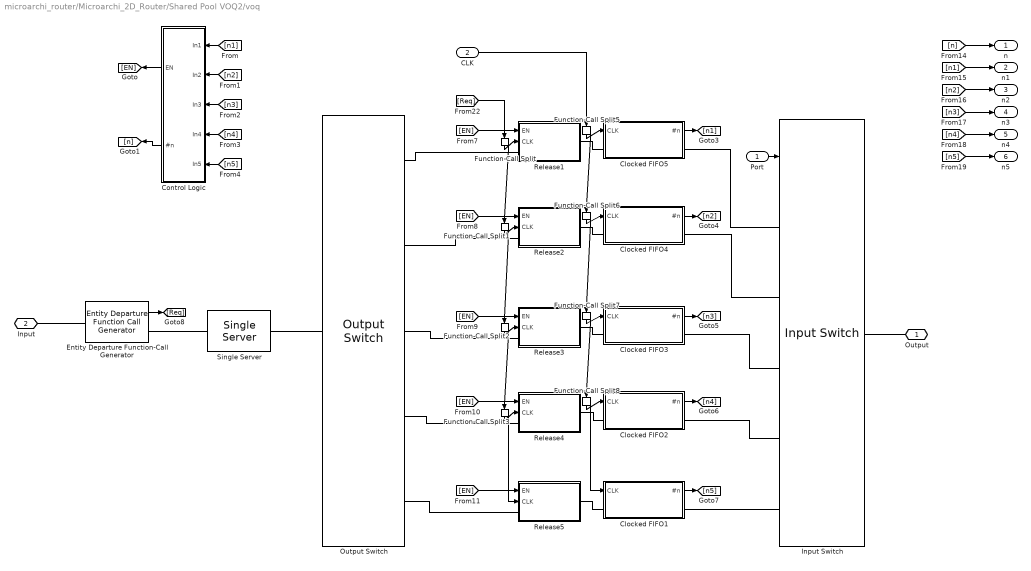
== system microarchi_router/Microarchi_2D_Router/Shared Pool VOQ2/voq ==
  Port : Inport
  CLK : Inport  Port=2
  Clocked FIFO1 : Subsystem  mask{E=0, S=0, F=C}
      mask prompts: E "Clock Period (s)"; S "Standard Deviation"; F "FIFO capacity"
  Clocked FIFO2 : Subsystem  mask{E=0, S=0, F=C}
      mask prompts: E "Clock Period (s)"; S "Standard Deviation"; F "FIFO capacity"
  Clocked FIFO3 : Subsystem  mask{E=0, S=0, F=C}
      mask prompts: E "Clock Period (s)"; S "Standard Deviation"; F "FIFO capacity"
  Clocked FIFO4 : Subsystem  mask{E=0, S=0, F=C}
      mask prompts: E "Clock Period (s)"; S "Standard Deviation"; F "FIFO capacity"
  Clocked FIFO5 : Subsystem  mask{E=0, S=0, F=C}
      mask prompts: E "Clock Period (s)"; S "Standard Deviation"; F "FIFO capacity"
  Control Logic : Subsystem  TreatAsAtomicUnit=on
  Entity Departure Function-Call Generator : EntityDepartureFunctionCallGenerator
  Function-Call Split{,1..3,5..8} (8 alike) : FunctionCallSplit
  Input Switch : InputSwitch  NumberInputPorts=5  SwitchingCriterion=From signal port p
  Output Switch : OutputSwitch  NumberOutputPorts=5  SwitchingCriterion=From attribute  AttributeName=RT
  Release1 : Subsystem
  Release2 : Subsystem
  Release3 : Subsystem
  Release4 : Subsystem
  Release5 : Subsystem
  Single Server : SingleServer  ServiceTime=0
  Output : PMIOPort  Port=1  Side=Right
  Input : PMIOPort  Port=2  Side=Left
  n : Outport
  n1 : Outport  Port=2
  n2 : Outport  Port=3
  n3 : Outport  Port=4
  n4 : Outport  Port=5
  n5 : Outport  Port=6
  wires:
  Port/1 -> Input Switch/1
  [n1] -> Control Logic/1(In1)
  [n2] -> Control Logic/2(In2)
  [n3] -> Control Logic/3(In3)
  [n5] -> Control Logic/5(In5)
  [n4] -> Control Logic/4(In4)
  Control Logic/1(EN) -> [EN]
  Control Logic/2(#n) -> [n]
  Clocked FIFO5/1(#n) -> [n1]
  Clocked FIFO4/1(#n) -> [n2]
  Clocked FIFO3/1(#n) -> [n3]
  Clocked FIFO2/1(#n) -> [n4]
  Clocked FIFO1/1(#n) -> [n5]
  [EN] -> Release5/1(EN)
  [EN] -> Release4/1(EN)
  [EN] -> Release3/1(EN)
  [EN] -> Release2/1(EN)
  [EN] -> Release1/1(EN)
  [n] -> n/1
  [n1] -> n1/1
  [n2] -> n2/1
  [n3] -> n3/1
  [n4] -> n4/1
  [n5] -> n5/1
  Entity Departure Function-Call Generator/1 -> [Req]
  Function-Call Split8/1 -> Clocked FIFO2/1(CLK)
  Function-Call Split7/2 -> Function-Call Split8/1
  Function-Call Split7/1 -> Clocked FIFO3/1(CLK)
  Function-Call Split6/2 -> Function-Call Split7/1
  Function-Call Split6/1 -> Clocked FIFO4/1(CLK)
  Function-Call Split5/2 -> Function-Call Split6/1
  Function-Call Split5/1 -> Clocked FIFO5/1(CLK)
  CLK/1 -> Function-Call Split5/1
  Function-Call Split/1 -> Release1/2(CLK)
  Function-Call Split1/1 -> Release2/2(CLK)
  Function-Call Split2/1 -> Release3/2(CLK)
  Function-Call Split3/1 -> Release4/2(CLK)
  Function-Call Split2/2 -> Function-Call Split3/1
  Function-Call Split1/2 -> Function-Call Split2/1
  Function-Call Split/2 -> Function-Call Split1/1
  [Req] -> Function-Call Split/1
  Function-Call Split8/2 -> Clocked FIFO1/1(CLK)
  Function-Call Split3/2 -> Release5/2(CLK)
  connections:
  Clocked FIFO5/LConn1 -- Release1/RConn1
  Input/RConn1 -- Entity Departure Function-Call Generator/LConn1
  Release3/RConn1 -- Clocked FIFO3/LConn1
  Release4/RConn1 -- Clocked FIFO2/LConn1
  Release2/RConn1 -- Clocked FIFO4/LConn1
  Release3/LConn1 -- Output Switch/RConn3
  Release2/LConn1 -- Output Switch/RConn2
  Release4/LConn1 -- Output Switch/RConn4
  Output Switch/RConn1 -- Release1/LConn1
  Input Switch/RConn1 -- Output/RConn1
  Release5/RConn1 -- Clocked FIFO1/LConn1
  Release5/LConn1 -- Output Switch/RConn5
  Clocked FIFO5/RConn1 -- Input Switch/LConn1
  Clocked FIFO4/RConn1 -- Input Switch/LConn2
  Clocked FIFO3/RConn1 -- Input Switch/LConn3
  Clocked FIFO2/RConn1 -- Input Switch/LConn4
  Clocked FIFO1/RConn1 -- Input Switch/LConn5
  Entity Departure Function-Call Generator/RConn1 -- Single Server/LConn1
  Single Server/RConn1 -- Output Switch/LConn1

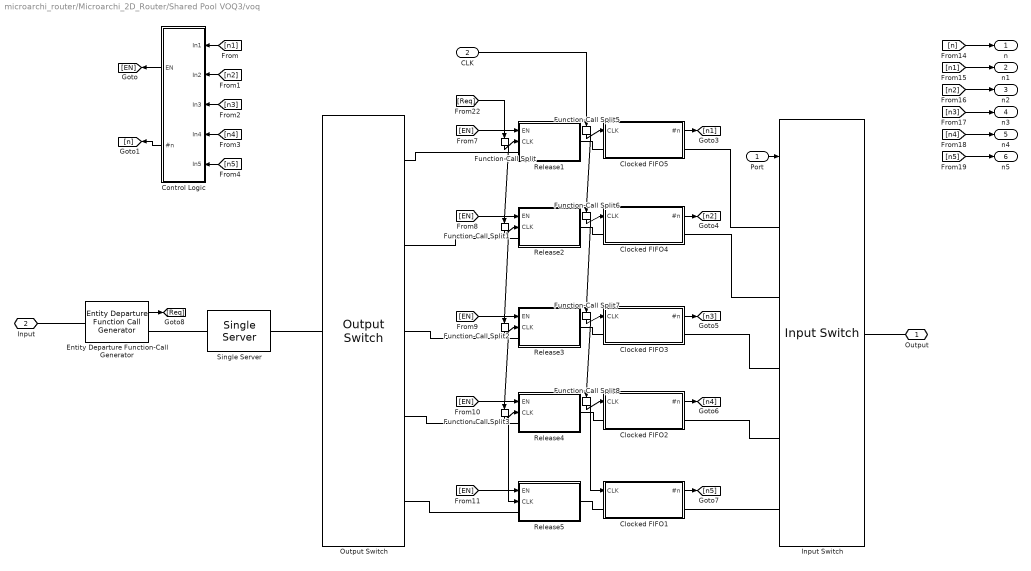
== system microarchi_router/Microarchi_2D_Router/Shared Pool VOQ3/voq ==
  Port : Inport
  CLK : Inport  Port=2
  Clocked FIFO1 : Subsystem  mask{E=0, S=0, F=C}
      mask prompts: E "Clock Period (s)"; S "Standard Deviation"; F "FIFO capacity"
  Clocked FIFO2 : Subsystem  mask{E=0, S=0, F=C}
      mask prompts: E "Clock Period (s)"; S "Standard Deviation"; F "FIFO capacity"
  Clocked FIFO3 : Subsystem  mask{E=0, S=0, F=C}
      mask prompts: E "Clock Period (s)"; S "Standard Deviation"; F "FIFO capacity"
  Clocked FIFO4 : Subsystem  mask{E=0, S=0, F=C}
      mask prompts: E "Clock Period (s)"; S "Standard Deviation"; F "FIFO capacity"
  Clocked FIFO5 : Subsystem  mask{E=0, S=0, F=C}
      mask prompts: E "Clock Period (s)"; S "Standard Deviation"; F "FIFO capacity"
  Control Logic : Subsystem  TreatAsAtomicUnit=on
  Entity Departure Function-Call Generator : EntityDepartureFunctionCallGenerator
  Function-Call Split{,1..3,5..8} (8 alike) : FunctionCallSplit
  Input Switch : InputSwitch  NumberInputPorts=5  SwitchingCriterion=From signal port p
  Output Switch : OutputSwitch  NumberOutputPorts=5  SwitchingCriterion=From attribute  AttributeName=RT
  Release1 : Subsystem
  Release2 : Subsystem
  Release3 : Subsystem
  Release4 : Subsystem
  Release5 : Subsystem
  Single Server : SingleServer  ServiceTime=0
  Output : PMIOPort  Port=1  Side=Right
  Input : PMIOPort  Port=2  Side=Left
  n : Outport
  n1 : Outport  Port=2
  n2 : Outport  Port=3
  n3 : Outport  Port=4
  n4 : Outport  Port=5
  n5 : Outport  Port=6
  wires:
  Function-Call Split3/2 -> Release5/2(CLK)
  Function-Call Split8/2 -> Clocked FIFO1/1(CLK)
  [Req] -> Function-Call Split/1
  Function-Call Split/2 -> Function-Call Split1/1
  Function-Call Split1/2 -> Function-Call Split2/1
  Function-Call Split2/2 -> Function-Call Split3/1
  Function-Call Split3/1 -> Release4/2(CLK)
  Function-Call Split2/1 -> Release3/2(CLK)
  Function-Call Split1/1 -> Release2/2(CLK)
  Function-Call Split/1 -> Release1/2(CLK)
  CLK/1 -> Function-Call Split5/1
  Function-Call Split5/1 -> Clocked FIFO5/1(CLK)
  Function-Call Split5/2 -> Function-Call Split6/1
  Function-Call Split6/1 -> Clocked FIFO4/1(CLK)
  Function-Call Split6/2 -> Function-Call Split7/1
  Function-Call Split7/1 -> Clocked FIFO3/1(CLK)
  Function-Call Split7/2 -> Function-Call Split8/1
  Function-Call Split8/1 -> Clocked FIFO2/1(CLK)
  Entity Departure Function-Call Generator/1 -> [Req]
  [n5] -> n5/1
  [n4] -> n4/1
  [n3] -> n3/1
  [n2] -> n2/1
  [n1] -> n1/1
  [n] -> n/1
  [EN] -> Release1/1(EN)
  [EN] -> Release2/1(EN)
  [EN] -> Release3/1(EN)
  [EN] -> Release4/1(EN)
  [EN] -> Release5/1(EN)
  Clocked FIFO1/1(#n) -> [n5]
  Clocked FIFO2/1(#n) -> [n4]
  Clocked FIFO3/1(#n) -> [n3]
  Clocked FIFO4/1(#n) -> [n2]
  Clocked FIFO5/1(#n) -> [n1]
  Control Logic/2(#n) -> [n]
  Control Logic/1(EN) -> [EN]
  [n4] -> Control Logic/4(In4)
  [n5] -> Control Logic/5(In5)
  [n3] -> Control Logic/3(In3)
  [n2] -> Control Logic/2(In2)
  [n1] -> Control Logic/1(In1)
  Port/1 -> Input Switch/1
  connections:
  Single Server/RConn1 -- Output Switch/LConn1
  Entity Departure Function-Call Generator/RConn1 -- Single Server/LConn1
  Clocked FIFO1/RConn1 -- Input Switch/LConn5
  Clocked FIFO2/RConn1 -- Input Switch/LConn4
  Clocked FIFO3/RConn1 -- Input Switch/LConn3
  Clocked FIFO4/RConn1 -- Input Switch/LConn2
  Clocked FIFO5/RConn1 -- Input Switch/LConn1
  Release5/LConn1 -- Output Switch/RConn5
  Release5/RConn1 -- Clocked FIFO1/LConn1
  Input Switch/RConn1 -- Output/RConn1
  Output Switch/RConn1 -- Release1/LConn1
  Release4/LConn1 -- Output Switch/RConn4
  Release2/LConn1 -- Output Switch/RConn2
  Release3/LConn1 -- Output Switch/RConn3
  Release2/RConn1 -- Clocked FIFO4/LConn1
  Release4/RConn1 -- Clocked FIFO2/LConn1
  Release3/RConn1 -- Clocked FIFO3/LConn1
  Input/RConn1 -- Entity Departure Function-Call Generator/LConn1
  Clocked FIFO5/LConn1 -- Release1/RConn1

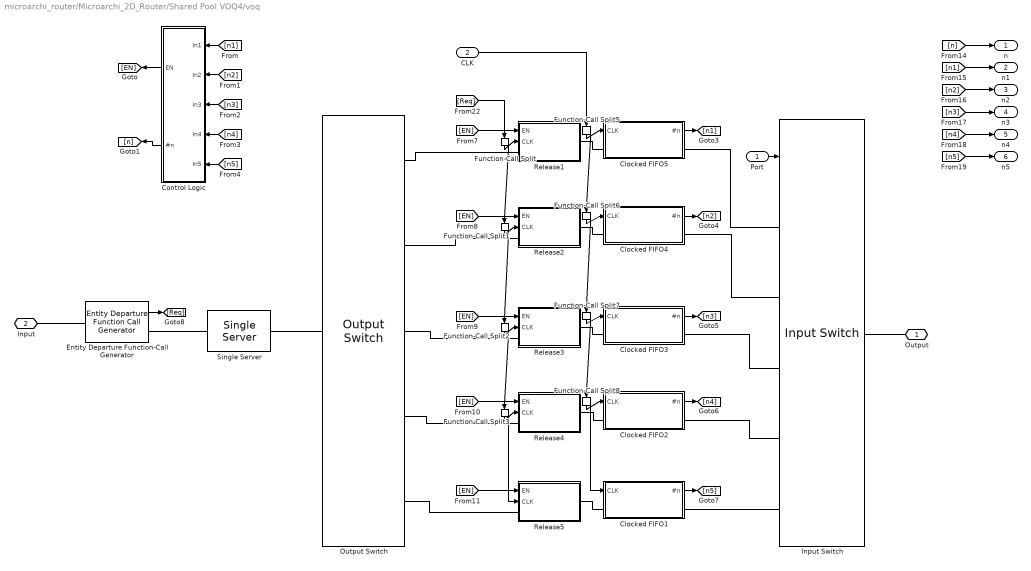
== system microarchi_router/Microarchi_2D_Router/Shared Pool VOQ4/voq ==
  Port : Inport
  CLK : Inport  Port=2
  Clocked FIFO1 : Subsystem  mask{E=0, S=0, F=C}
      mask prompts: E "Clock Period (s)"; S "Standard Deviation"; F "FIFO capacity"
  Clocked FIFO2 : Subsystem  mask{E=0, S=0, F=C}
      mask prompts: E "Clock Period (s)"; S "Standard Deviation"; F "FIFO capacity"
  Clocked FIFO3 : Subsystem  mask{E=0, S=0, F=C}
      mask prompts: E "Clock Period (s)"; S "Standard Deviation"; F "FIFO capacity"
  Clocked FIFO4 : Subsystem  mask{E=0, S=0, F=C}
      mask prompts: E "Clock Period (s)"; S "Standard Deviation"; F "FIFO capacity"
  Clocked FIFO5 : Subsystem  mask{E=0, S=0, F=C}
      mask prompts: E "Clock Period (s)"; S "Standard Deviation"; F "FIFO capacity"
  Control Logic : Subsystem  TreatAsAtomicUnit=on
  Entity Departure Function-Call Generator : EntityDepartureFunctionCallGenerator
  Function-Call Split{,1..3,5..8} (8 alike) : FunctionCallSplit
  Input Switch : InputSwitch  NumberInputPorts=5  SwitchingCriterion=From signal port p
  Output Switch : OutputSwitch  NumberOutputPorts=5  SwitchingCriterion=From attribute  AttributeName=RT
  Release1 : Subsystem
  Release2 : Subsystem
  Release3 : Subsystem
  Release4 : Subsystem
  Release5 : Subsystem
  Single Server : SingleServer  ServiceTime=0
  Output : PMIOPort  Port=1  Side=Right
  Input : PMIOPort  Port=2  Side=Left
  n : Outport
  n1 : Outport  Port=2
  n2 : Outport  Port=3
  n3 : Outport  Port=4
  n4 : Outport  Port=5
  n5 : Outport  Port=6
  wires:
  Port/1 -> Input Switch/1
  [n1] -> Control Logic/1(In1)
  [n2] -> Control Logic/2(In2)
  [n3] -> Control Logic/3(In3)
  [n5] -> Control Logic/5(In5)
  [n4] -> Control Logic/4(In4)
  Control Logic/1(EN) -> [EN]
  Control Logic/2(#n) -> [n]
  Clocked FIFO5/1(#n) -> [n1]
  Clocked FIFO4/1(#n) -> [n2]
  Clocked FIFO3/1(#n) -> [n3]
  Clocked FIFO2/1(#n) -> [n4]
  Clocked FIFO1/1(#n) -> [n5]
  [EN] -> Release5/1(EN)
  [EN] -> Release4/1(EN)
  [EN] -> Release3/1(EN)
  [EN] -> Release2/1(EN)
  [EN] -> Release1/1(EN)
  [n] -> n/1
  [n1] -> n1/1
  [n2] -> n2/1
  [n3] -> n3/1
  [n4] -> n4/1
  [n5] -> n5/1
  Entity Departure Function-Call Generator/1 -> [Req]
  Function-Call Split8/1 -> Clocked FIFO2/1(CLK)
  Function-Call Split7/2 -> Function-Call Split8/1
  Function-Call Split7/1 -> Clocked FIFO3/1(CLK)
  Function-Call Split6/2 -> Function-Call Split7/1
  Function-Call Split6/1 -> Clocked FIFO4/1(CLK)
  Function-Call Split5/2 -> Function-Call Split6/1
  Function-Call Split5/1 -> Clocked FIFO5/1(CLK)
  CLK/1 -> Function-Call Split5/1
  Function-Call Split/1 -> Release1/2(CLK)
  Function-Call Split1/1 -> Release2/2(CLK)
  Function-Call Split2/1 -> Release3/2(CLK)
  Function-Call Split3/1 -> Release4/2(CLK)
  Function-Call Split2/2 -> Function-Call Split3/1
  Function-Call Split1/2 -> Function-Call Split2/1
  Function-Call Split/2 -> Function-Call Split1/1
  [Req] -> Function-Call Split/1
  Function-Call Split8/2 -> Clocked FIFO1/1(CLK)
  Function-Call Split3/2 -> Release5/2(CLK)
  connections:
  Clocked FIFO5/LConn1 -- Release1/RConn1
  Input/RConn1 -- Entity Departure Function-Call Generator/LConn1
  Release3/RConn1 -- Clocked FIFO3/LConn1
  Release4/RConn1 -- Clocked FIFO2/LConn1
  Release2/RConn1 -- Clocked FIFO4/LConn1
  Release3/LConn1 -- Output Switch/RConn3
  Release2/LConn1 -- Output Switch/RConn2
  Release4/LConn1 -- Output Switch/RConn4
  Output Switch/RConn1 -- Release1/LConn1
  Input Switch/RConn1 -- Output/RConn1
  Release5/RConn1 -- Clocked FIFO1/LConn1
  Release5/LConn1 -- Output Switch/RConn5
  Clocked FIFO5/RConn1 -- Input Switch/LConn1
  Clocked FIFO4/RConn1 -- Input Switch/LConn2
  Clocked FIFO3/RConn1 -- Input Switch/LConn3
  Clocked FIFO2/RConn1 -- Input Switch/LConn4
  Clocked FIFO1/RConn1 -- Input Switch/LConn5
  Entity Departure Function-Call Generator/RConn1 -- Single Server/LConn1
  Single Server/RConn1 -- Output Switch/LConn1

== system microarchi_router/Microarchi_2D_Router/Shared Pool VOQ/voq/Clocked FIFO1 ==
  CLK : Inport
  FIFO Queue : FIFOQueue  Capacity=F  StatNumberInBlock=on
      settings: OutputPortMap=o1
  Release Gate : ReleaseGate  OpenGateUpon=Function call from port fcn
  Single Server : SingleServer  ServiceTime=0
  Input : PMIOPort  Port=1  Side=Left
  Output : PMIOPort  Port=2  Side=Right
  #n : Outport
  wires:
  FIFO Queue/1 -> #n/1
  CLK/1 -> Release Gate/1
  connections:
  FIFO Queue/RConn1 -- Single Server/LConn1
  Single Server/RConn1 -- Release Gate/LConn1
  Release Gate/RConn1 -- Output/RConn1
  FIFO Queue/LConn1 -- Input/RConn1

== system microarchi_router/Microarchi_2D_Router/Shared Pool VOQ/voq/Clocked FIFO2 ==
  CLK : Inport
  FIFO Queue : FIFOQueue  Capacity=F  StatNumberInBlock=on
      settings: OutputPortMap=o1
  Release Gate : ReleaseGate  OpenGateUpon=Function call from port fcn
  Single Server : SingleServer  ServiceTime=0
  Input : PMIOPort  Port=1  Side=Left
  Output : PMIOPort  Port=2  Side=Right
  #n : Outport
  wires:
  CLK/1 -> Release Gate/1
  FIFO Queue/1 -> #n/1
  connections:
  FIFO Queue/LConn1 -- Input/RConn1
  Release Gate/RConn1 -- Output/RConn1
  Single Server/RConn1 -- Release Gate/LConn1
  FIFO Queue/RConn1 -- Single Server/LConn1

== system microarchi_router/Microarchi_2D_Router/Shared Pool VOQ/voq/Clocked FIFO3 ==
  CLK : Inport
  FIFO Queue : FIFOQueue  Capacity=F  StatNumberInBlock=on
      settings: OutputPortMap=o1
  Release Gate : ReleaseGate  OpenGateUpon=Function call from port fcn
  Single Server : SingleServer  ServiceTime=0
  Input : PMIOPort  Port=1  Side=Left
  Output : PMIOPort  Port=2  Side=Right
  #n : Outport
  wires:
  FIFO Queue/1 -> #n/1
  CLK/1 -> Release Gate/1
  connections:
  FIFO Queue/RConn1 -- Single Server/LConn1
  Single Server/RConn1 -- Release Gate/LConn1
  Release Gate/RConn1 -- Output/RConn1
  FIFO Queue/LConn1 -- Input/RConn1

== system microarchi_router/Microarchi_2D_Router/Shared Pool VOQ/voq/Clocked FIFO4 ==
  CLK : Inport
  FIFO Queue : FIFOQueue  Capacity=F  StatNumberInBlock=on
      settings: OutputPortMap=o1
  Release Gate : ReleaseGate  OpenGateUpon=Function call from port fcn
  Single Server : SingleServer  ServiceTime=0
  Input : PMIOPort  Port=1  Side=Left
  Output : PMIOPort  Port=2  Side=Right
  #n : Outport
  wires:
  CLK/1 -> Release Gate/1
  FIFO Queue/1 -> #n/1
  connections:
  FIFO Queue/LConn1 -- Input/RConn1
  Release Gate/RConn1 -- Output/RConn1
  Single Server/RConn1 -- Release Gate/LConn1
  FIFO Queue/RConn1 -- Single Server/LConn1

== system microarchi_router/Microarchi_2D_Router/Shared Pool VOQ/voq/Clocked FIFO5 ==
  CLK : Inport
  FIFO Queue : FIFOQueue  Capacity=F  StatNumberInBlock=on
      settings: OutputPortMap=o1
  Release Gate : ReleaseGate  OpenGateUpon=Function call from port fcn
  Single Server : SingleServer  ServiceTime=0
  Input : PMIOPort  Port=1  Side=Left
  Output : PMIOPort  Port=2  Side=Right
  #n : Outport
  wires:
  FIFO Queue/1 -> #n/1
  CLK/1 -> Release Gate/1
  connections:
  FIFO Queue/RConn1 -- Single Server/LConn1
  Single Server/RConn1 -- Release Gate/LConn1
  Release Gate/RConn1 -- Output/RConn1
  FIFO Queue/LConn1 -- Input/RConn1
